simulink model "AdaptiveOscillators"  (R2019b)
settings: Solver=FixedStepAuto  StartTime=0.0  StopTime=N*T  FixedStep=tsamp  MaxStep=0.01  RelTol=1e-3
values from neighbouring files (symbols this model uses):
  alpha_r = 0.35    [AO_Oscillators.m]    (also in PoolofAdaptiveOscillatorsThree.m)
  eta = 2    [AO_Oscillators.m]    (also in PoolofAdaptiveOscillatorsThree.m = 1)
  omega_r = 2*pi/T    (= 5.02654824574)    [AO_Oscillators.m]    (also in PoolofAdaptiveOscillatorsThree.m)
  v_omega = 13    [AO_Oscillators.m]    (also in PoolofAdaptiveOscillatorsThree.m = 2)
  v_phi = sqrt(24.2*v_omega)    [AO_Oscillators.m]    (also in PoolofAdaptiveOscillatorsThree.m = 2)
settings Model: Creator=dell  LastModifiedBy=dell

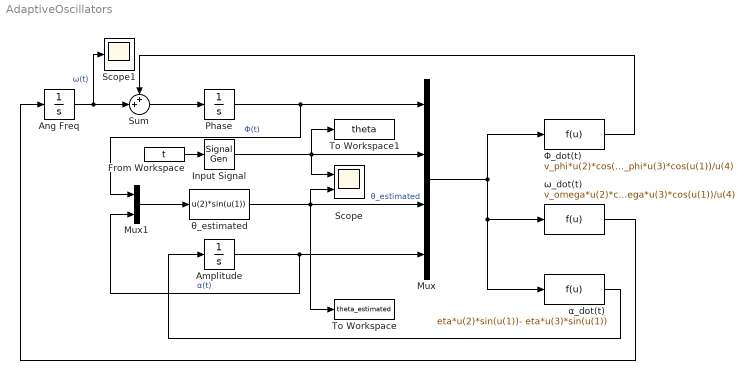
== system AdaptiveOscillators ==
  Amplitude : Integrator  InitialCondition=0.1  ContinuousStateAttributes='Amplitude'
  Ang Freq : Integrator  ContinuousStateAttributes='AngularFrequency'
  From Workspace : FromWorkspace  VariableName=t  SampleTime=0
  Input Signal : SignalGenerator  TimeSource=Use external signal  Amplitude=alpha_r  Frequency=omega_r  Units=rad/sec
  Mux : Mux
  Mux1 : Mux  Inputs=2
  Phase : Integrator  InitialCondition=0.001  ContinuousStateAttributes='Phase'
  Scope : Scope  NumInputPorts=2
  Scope1 : Scope
  Sum : Sum  Inputs=++|
  To Workspace : ToWorkspace  VariableName=theta_estimated  SaveFormat=Timeseries  SampleTime=-1
  To Workspace1 : ToWorkspace  VariableName=theta  SaveFormat=Timeseries  SampleTime=-1
  Φ_dot(t) : Fcn  Expr=v_phi*u(2)*cos(u(1))/u(4) - v_phi*u(3)*cos(u(1))/u(4)
  α_dot(t) : Fcn  Expr=eta*u(2)*sin(u(1))- eta*u(3)*sin(u(1))
  θ_estimated : Fcn  Expr=u(2)*sin(u(1))
  ω_dot(t) : Fcn  Expr=v_omega*u(2)*cos(u(1))/u(4) - v_omega*u(3)*cos(u(1))/u(4)
  wires:
  Mux1/1 -> θ_estimated/1
  θ_estimated/1 -> To Workspace/1, Mux/3, Scope/2  "θ_estimated"
  Phase/1 -> Mux1/1, Mux/1  "Φ(t)"
  Amplitude/1 -> Mux1/2, Mux/4  "α(t)"
  Mux/1 -> ω_dot(t)/1, α_dot(t)/1, Φ_dot(t)/1
  Ang Freq/1 -> Scope1/1, Sum/2  "ω(t)"
  Φ_dot(t)/1 -> Sum/1
  ω_dot(t)/1 -> Ang Freq/1
  α_dot(t)/1 -> Amplitude/1
  Sum/1 -> Phase/1
  Input Signal/1 -> To Workspace1/1, Scope/1, Mux/2
  From Workspace/1 -> Input Signal/1
